simulink model "Lab6_1_2"  (R2020b)
settings: Solver=VariableStepAuto  StartTime=0.0  StopTime=10.0  RelTol=1e-3
undefined symbols (not defined in the file): A, h, ym
settings Model: Creator=Maciek  LastModifiedBy=Maciek

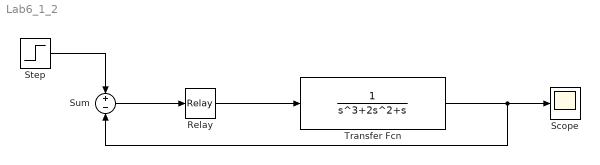
== system Lab6_1_2 ==
  Relay : Relay  OnSwitchValue=h  OffSwitchValue=-h  OnOutputValue=ym  OffOutputValue=-ym
  Scope : Scope
  Step : Step  After=A  SampleTime=0
  Sum : Sum  Inputs=+-
  Transfer Fcn : TransferFcn  Denominator=[1 2 1 0]
  wires:
  Transfer Fcn/1 -> Sum/2, Scope/1
  Sum/1 -> Relay/1
  Relay/1 -> Transfer Fcn/1
  Step/1 -> Sum/1
